simulink model "Cruise_Model_V10_hmm"  (R2024a)
settings: Solver=ode23t  StartTime=0.0  StopTime=20  RelTol=1e-3
values from neighbouring files (symbols this model uses):
  K = [-3.60668197653e-15 -4.8519082962e-07 3.58300531153e-06 -0.0035102270316 8.3861852137e-07 3.06276240474 1.22104661107e-16 -0.00351023001393 8.38621571888e-07 3.0627647777 2.01711556188e-16 0.00352147083436 ... (11970 elements, 19x9x70)]    [alexisignoringme2.mat]    (also in alexisignoringme3.mat = [-2.3054870934e-16 -3.29424508508e-08 -2.01640092228e-07 -0.; alexisignoringme4.mat = [-2.3054870934e-16 -3.29424508508e-08 -2.01640092228e-07 -0.; plotLQI_LQR_Comparison.m = Kf(:,:,idx(i)); selectQRfull.m = createGainMat(sysMat, 'QRValsLQR', 'trimUAM1'))
  missionruntime =     [alexisignoringme2.mat]    (also in alexisignoringme3.mat; alexisignoringme4.mat; selectQRfull.m = rmfield(missionruntime, 'rotorTilt'))
  referenceGeo =     [alexisignoringme2.mat]    (also in alexisignoringme3.mat; alexisignoringme4.mat)
  U = [2.18842852529e-05 -1.75359463768e-06 7.65324951435e-07 376.143045818 0 0 0 376.144413812 0 0 0 376.143045818 ... (1330 elements, 19x70)]    [alexisignoringme2.mat]    (also in alexisignoringme3.mat = [-1.76080437445e-06 1.51055858734e-07 -7.54037213995e-08 346; createPlots.m = trim.U; selectQRfull.m = reshape(trim.U,size(trim.U,1),[]); trimCost.m = [Z(7:9)' Z(10) 0 rpitch 0              Z(11) 0 rpitch 0     )
  X = [0.00351655091712 0 -9.99999601592 0 0 0 -4.86374081337e-08 -4.19859407075e-06 -3.62256781384e-09 0.00728108667364 0 -9.23082547646 ... (630 elements, 9x70)]    [alexisignoringme2.mat]    (also in alexisignoringme3.mat = [0.00351658839646 0 -9.99999599468 0 0 0 2.7327442949e-09 -4; alexisignoringme4.mat = [20 0 0 0 0 0 0 0 0]; createPlots.m = trim.X; selectQRfull.m = reshape(trim.X,size(trim.X,1),[]))
  Xe = [24.9700402552 0 -1.16861141766 0 0 0 1.12298779449e-07 -0.0450942805758 0.321650208764]    [alexisignoringme2.mat]    (also in alexisignoringme3.mat = [24.9726490597 0 -1.16896704065 0 0 0 -8.24889531393e-07 -0.; alexisignoringme4.mat = [24.9726490597 0 -1.16896704065 0 0 0 -8.24889531393e-07 0.0; plotLQI_LQR_Comparison.m = X(:,idx(i)+1); testGains.m = X(:,idx+1))
  Xes = [24.97004028 0 -1.16861086303 0 0 0 -5.01724449102e-07 -0.0450956248882 0.321650295301]    [alexisignoringme2.mat]    (also in alexisignoringme3.mat = [0.00351658839646 0 -9.99999599468 0 0 0 2.7327442949e-09 -4; alexisignoringme4.mat = [0 0 -1.11199998303 0 0 0 -1.38069247376e-09 1.48137256273e-; plotLQI_LQR_Comparison.m = X(:,idx(i)); selectQRfull.m = X(:,1))
undefined symbols (not defined in the file or in its folder): F, Light, MIL
libraries: slpidlib x14, aerolibwind2 x8, aerolibatmos2 x4, shared6dof x1
(part 3 of 3)

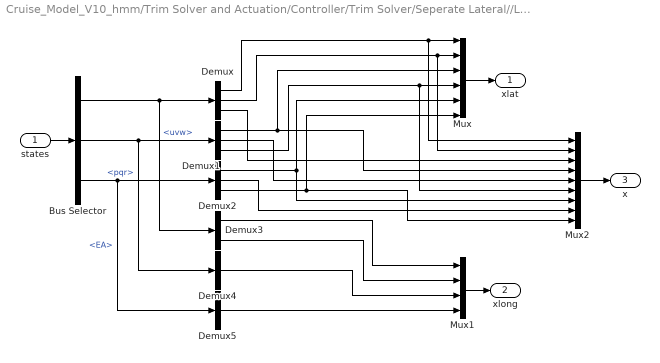
== system Cruise_Model_V10_hmm/Trim Solver and Actuation/Controller/Trim Solver/Seperate Lateral//Longitudinal ==
  states : Inport
  Bus Selector : BusSelector  OutputSignals=uvw,pqr,EA
  Demux{,1..5} (6 alike) : Demux  Outputs=3
  Mux : Mux  Inputs=6
  Mux1 : Mux
  Mux2 : Mux  Inputs=9
  xlat : Outport
  xlong : Outport  Port=2
  x : Outport  Port=3
  wires:
  states/1 -> Bus Selector/1
  Mux/1 -> xlat/1
  Mux1/1 -> xlong/1
  Bus Selector/1 -> Demux/1, Demux3/1  "<uvw>"
  Bus Selector/2 -> Demux1/1, Demux4/1  "<pqr>"
  Bus Selector/3 -> Demux5/1, Demux2/1  "<EA>"
  Demux/1 -> Mux2/1, Mux/1
  Demux/2 -> Mux2/2, Mux/2
  Demux1/1 -> Mux2/4, Mux/3
  Demux1/3 -> Mux2/6, Mux/4
  Demux2/1 -> Mux2/7, Mux/5
  Demux2/3 -> Mux2/9, Mux/6
  Demux3/1 -> Mux1/1
  Demux3/3 -> Mux1/2
  Demux4/2 -> Mux1/3
  Demux5/2 -> Mux1/4
  Mux2/1 -> x/1
  Demux/3 -> Mux2/3
  Demux1/2 -> Mux2/5
  Demux2/2 -> Mux2/8

== system Cruise_Model_V10_hmm/Trim Solver and Actuation/Controller/PID_GBDP_withThrust/Altitude Control Path/Step demand for testing ==
  In1 : Inport
  Mux1 : Mux  Inputs=2
  Scope2 : Scope
  Scope4 : Scope
  Step1 : Step  Time=60  Before=-500  After=-490  SampleTime=0
  Step2 : Step  Time=80  After=-10  SampleTime=0
  Step3 : Step  Time=120  After=20  SampleTime=0
  Step4 : Step  Time=120  After=20  SampleTime=0
  Sum : Sum  Inputs=++++
  To Workspace : ToWorkspace  VariableName=altitudeResponse  SaveFormat=Timeseries  SampleTime=-1
  Out1 : Outport
  wires:
  Step3/1 -> Sum/3
  Mux1/1 -> To Workspace/1, Scope4/1
  Sum/1 -> Out1/1, Mux1/1
  Step4/1 -> Sum/4
  Step1/1 -> Sum/1
  In1/1 -> Mux1/2, Scope2/1
  Step2/1 -> Sum/2

== system Cruise_Model_V10_hmm/Trim Solver and Actuation/Controller/PID_GBDP_withThrust/Course Angle Control Path/Step demand for testing2 ==
  Va : Inport
  Mux1 : Mux  Inputs=2
  Scope2 : Scope
  Scope4 : Scope
  Step1 : Step  Time=60  Before=0.1  After=0.2  SampleTime=0
  Step2 : Step  Time=80  After=-0.4  SampleTime=0
  Step3 : Step  Time=120  After=-0.2  SampleTime=0
  Step4 : Step  Time=100  After=0.6  SampleTime=0
  Step5 : Step  Time=140  After=-0.4  SampleTime=0
  Sum : Sum  Inputs=+++++
  To Workspace : ToWorkspace  VariableName=headingAngleResponse  SaveFormat=Timeseries  SampleTime=-1
  Out1 : Outport
  wires:
  Step5/1 -> Sum/5
  Step3/1 -> Sum/3
  Mux1/1 -> To Workspace/1, Scope4/1
  Sum/1 -> Out1/1, Mux1/1
  Step4/1 -> Sum/4
  Step1/1 -> Sum/1
  Va/1 -> Mux1/2, Scope2/1
  Step2/1 -> Sum/2

== system Cruise_Model_V10_hmm/Trim Solver and Actuation/Controller/PID_GBDP_withThrust/Subsystem/Step demand for testing1 ==
  Va : Inport
  Mux1 : Mux  Inputs=2
  Scope2 : Scope
  Scope4 : Scope
  Step1 : Step  Time=60  Before=25  After=31  SampleTime=0
  Step2 : Step  Time=80  After=-3  SampleTime=0
  Step3 : Step  Time=120  After=-5  SampleTime=0
  Step4 : Step  Time=100  After=8  SampleTime=0
  Step5 : Step  Time=140  After=-2  SampleTime=0
  Sum : Sum  Inputs=+++++
  To Workspace : ToWorkspace  VariableName=airspeedResponse  SaveFormat=Timeseries  SampleTime=-1
  Out1 : Outport
  wires:
  Step2/1 -> Sum/2
  Va/1 -> Scope2/1, Mux1/2
  Step1/1 -> Sum/1
  Step4/1 -> Sum/4
  Sum/1 -> Mux1/1, Out1/1
  Mux1/1 -> Scope4/1, To Workspace/1
  Step3/1 -> Sum/3
  Step5/1 -> Sum/5

== matlab function Cruise_Model_V10_hmm/Trim Solver and Actuation/Controller/Trim Solver/MATLAB Function2 ==
  data: idx output; uref output; Ue input; time input; mission parameter
function [idx, uref] = fcn(Ue, time, mission)

t = linspace(0, mission.secTime(end), size(Ue,2));
[~, idx] = min(abs(t - time));

uref = Ue(:,idx);

== matlab function Cruise_Model_V10_hmm/Aircraft Dynamics/Aerodynamic Forces and Moments/MATLAB Function ==
  data: Fb output; Mcg output; coeff input Bus: coeff; u input; alpha input; beta input; V input; rho input; X input; refGeo parameter; m parameter; thrust input; cg parameter
function [Fb,Mcg] = aeroDyn(coeff, u, alpha, beta, V, rho, X, refGeo, m, thrust, cg)
% Function aeroDyn simulates ....

%% Setting up intermediate variables
b = refGeo.bref;
S = refGeo.Sref;
c = refGeo.cref;

Q = 0.5*rho*V^2; % Dynamic pressure Q

ndc = c/(2*V);
ndb = b/(2*V);

%% Seperating vectors (BFR)
uvw = X(1:3); % Translational velocity vector
pqr = X(4:6); % Angular velocity vector
EA = X(7:end);

%% Handle Stall

%% Non-dimensional Aerodynamic Force Coefficients
% In wind axis
% Lift
CL = applyDeriv(coeff.CL0, coeff.CLa, coeff.CLb, coeff.CLn, 0, coeff.CLq, 0, u, alpha, beta, pqr, ndc);

% Drag 
CD = applyDeriv(coeff.CD0, coeff.CDa, coeff.CDb, coeff.CDn, 0, 0, 0, u, alpha, beta, pqr, ndc);

% Sideforce
CY = applyDeriv(0, coeff.CYa, coeff.CYb, coeff.CYn, coeff.CYp, 0, coeff.CYr, u, alpha, beta, pqr, ndb);

if abs(alpha) > 14.5*(pi/180)
    CL = 0;
    CD = coeff.CD0;
end

%% Rotate wind to body
Faw = [-max(CD,0); CY; -CL].*Q*S; % Force vector in the stability frame

Rwb = [cos(alpha)*cos(beta), -cos(alpha)*sin(beta), -sin(alpha);  
       sin(beta)           ,  cos(beta)           ,  0         ; 
       cos(beta)*sin(alpha), -sin(alpha)*sin(beta),  cos(alpha)];

Fab = Rwb*Faw; % aerodynamic force on body

%% Aerodynamic Moment about CG
% In Fb, with moments taken about the centre of gravity

% Roll
Cl = applyDeriv(0, coeff.Cla, coeff.Clb, coeff.Cln, coeff.Clp, 0, coeff.Clr, u, alpha, beta, pqr, ndb);

% Pitch
Cm = applyDeriv(coeff.Cm0, coeff.Cma, coeff.Cmb, coeff.Cmn, 0, coeff.Cmq, 0, u, alpha, beta, pqr, ndc);

% Yaw
Cn = applyDeriv(0, coeff.Cna, coeff.Cnb, coeff.Cnn, coeff.Cnp, 0, coeff.Cnr, u, alpha, beta, pqr, ndb);

if abs(alpha) > 20*(pi/180)
    Cm = 0;
end

Ma = [b*Cl; c*Cm; b*Cn].*Q*S;

%% Propulsion Effects
% Moment and forces induced by throttle
FTb = zeros(3, length(thrust.Tinit));
MTcg = zeros(3, length(thrust.Tinit));

for i = 1:length(thrust.Tinit)
    idx = length(coeff.CLn) + 1 + (i-1)*4; % index of thrust-deflection pairs for thrust objects
    FTt = [0      ; % Thrust in rotor plane
           0      ;
           -u(idx)];
    
    Rrb = transMatrix([u(idx+1) u(idx+2) u(idx+3)].*[1 1 1]); % rotation matrix from rotor plane to body, first converting to geometric axis

    FTb(:,i) = Rrb*FTt; % Rotate to body frame, switching from geometric to dynamic coordinates
    MTcg(:,i) = cross(thrust.xyz_tr(i,:) - cg, FTb(:,i));
end

FTb = sum(FTb,2);
MTcg = sum(MTcg,2);

% Gravity Effects
Fgb = [-9.81*sin(X(8))          ; % Body frame
        9.81*cos(X(8))*sin(X(7));
        9.81*cos(X(8))*cos(X(7))]*m; % ASSUMPTION: Constant Mass

%% Out
Rbe = body2earth(X(7), X(8), X(9));

Fb = FTb + Fgb + Fab;
Mcg = MTcg + Ma;

forces = [FTb; Fgb; Fab; Rbe*Fb];
aero = [CL; CD; Cm];
uvw_e = Rbe*X(1:3);

end

%% Extra functions

function C = applyDeriv(C0, Ca, Cb, Cn, Cp, Cq, Cr, u, alpha, beta, pqr, nd)
% function applyDeriv calculates the coefficient C from the derivatives C0,
% Ca, Cb, Cn wrt 0, alpha, beta and control (n), respectively.

    C_nc = C0 + Ca*alpha + Cb*beta + Cp*pqr(1)*nd + Cq*pqr(2)*nd + Cr*pqr(3)*nd; % lift coefficient no control
    
    C_c = (Cn.*u(1:length(Cn)))';

    C = C_nc + sum(C_c);

end

== matlab function Cruise_Model_V10_hmm/Trim Solver and Actuation/Controller/Trim Solver/MATLAB Function1 ==
  data: idx output; xref_lat output; Xe input; time input; mission parameter; xref_long output; xref output
function [idx, xref_lat, xref_long, xref] = fcn(Xe, time, mission)

t = linspace(0, mission.secTime(end), size(Xe,2));
[~, idx] = min(abs(t - time));

xref = Xe(:,idx);
xref_lat = xref([1 2 4 6 7 9]);
xref_long = xref([1 3 5 8]);

== matlab function Cruise_Model_V10_hmm/Trim Solver and Actuation/Controller/Trim Solver/MATLAB Function ==
  data: xref input; U output; idx input; K input
function U = fcn(xref, idx, K)

U = K(:,:,idx+1)*xref;
